simulink model "PEMFuelCellSystem_Before_v01"  (R2025b)
settings: Solver=VariableStepAuto  StartTime=0.0  StopTime=0.1  MaxStep=0.01  RelTol=1e-3  AbsTol=1e-3
model workspace: external: MATLAB File E:\agentwork_pemfc_cEGR_0519\04_Simulink物理网络模型\01_模型\RouteA_GasMixture_Derived\PEMFuelCellSystemWithACustomLibraryParameters.m (data not in the file)
undefined symbols (not defined in the file): anode_tube_D, cathode_tube_D, cegr_valve_max_area, cegr_valve_open_min_area, comp_rpm_TLU, coolant_num_layers, coolant_num_passes, coolant_tube_D, coolant_w_channels, env_p, env_T, env_yH20, env_yO2, radiator_air_area_fins, radiator_air_area_primary, radiator_eta_fin, radiator_N_tubes, radiator_rho, radiator_t_wall, radiator_tube_H, radiator_W, routeA_air_pid_Ki, routeA_air_pid_Kp, routeA_anode_inlet_pressure_MPa_abs, routeA_anode_purge_off_n2_mole_fraction, routeA_anode_purge_on_n2_mole_fraction, routeA_anode_recirculation_base_command, routeA_anode_recirculation_current_gain_A_inv, routeA_anode_rh_setpoint, routeA_cathode_humidifier_gain, routeA_cathode_rh_setpoint, routeA_compressor_cmd_direct, routeA_egr_control_Ki_area, routeA_egr_control_Kp_area, routeA_egr_target_input_mode_id, routeA_egr_valve_actuator_tau, routeA_egr_valve_area_direct, routeA_stack_temperature_set_C, routeA_target_egr_ratio_comp_in, routeA_target_mdot_comp_inlet, routeA_target_oer, routeA_target_p_ca_out_MPa, routeA_voltage_current_max_A, routeA_voltage_current_min_A, routeA_voltage_pi_Ki, routeA_voltage_pi_Kp, stack_area, stack_iL, stack_mea_rho, stack_num_cells, stack_num_channels, stack_t_gdl, stack_t_membrane, stack_w_channels, tank_yH2
libraries: fl_lib x63, FuelCell_lib x53, nesl_utility x42, slpidlib x5
(part 6 of 6)

== system PEMFuelCellSystem_Before_v01/System_Control_Observability/Electrical Load/Inputs/Power Demand ==
  From Workspace : FromWorkspace  VariableName=[drive_cycle_time, drive_cycle_power]
  PS Divide : fl_lib/Physical Signals/Functions/PS Divide
  PS-Simulink Converter : nesl_utility/PS-Simulink Converter  PhysicalDomain=network_engine_domain  SubClassName=ps_output  LeftPortType=input  RightPortType=output  PseudoPeriodic=off  Frequencies=[]  VectorFormat=1-D array  Unit=V  AffineConversion=off
  PS-Simulink Converter1 : nesl_utility/PS-Simulink Converter  PhysicalDomain=network_engine_domain  SubClassName=ps_output  LeftPortType=input  RightPortType=output  PseudoPeriodic=off  Frequencies=[]  VectorFormat=1-D array  Unit=A  AffineConversion=off
  Power Current Limit : fl_lib/Physical Signals/Nonlinear Operators/PS Saturation  upper_limit=routeA_voltage_current_max_A A  lower_limit=routeA_voltage_current_min_A A  ZeroCross=true
  Power kW to W : Gain  Gain=1000
  Simulink-PS Converter : nesl_utility/Simulink-PS Converter  PhysicalDomain=network_engine_domain  SubClassName=ps_input  LeftPortType=input  RightPortType=output  PseudoPeriodic=off  Frequencies=[]  NoiseDistribution=none  NoiseParameters=[]  Unit=W  AffineConversion=off  FilteringAndDerivatives=provide  SimscapeFilterOrder=1  InputFilterTimeConstant=0.001  UdotUserProvided=0
  i : PMIOPort  Side=Left
  v : PMIOPort  Port=2  Side=Left
  tag scope: i_stack=global, v_stack=global
  wires:
  PS-Simulink Converter1/1 -> [i_stack]  "routeA_power_current_cmd_limited_A"
  PS-Simulink Converter/1 -> [v_stack]
  From Workspace/1 -> Power kW to W/1
  Power kW to W/1 -> Simulink-PS Converter/1
  connections:
  PS-Simulink Converter1/LConn1 -- Power Current Limit/RConn1 -- i/RConn1
  v/RConn1 -- PS-Simulink Converter/LConn1 -- PS Divide/LConn2
  PS Divide/LConn1 -- Simulink-PS Converter/RConn1
  PS Divide/RConn1 -- Power Current Limit/LConn1

== system PEMFuelCellSystem_Before_v01/System_Control_Observability/Electrical Load/Inputs/Voltage Demand ==
  Current Command : nesl_utility/Simulink-PS Converter  PhysicalDomain=network_engine_domain  SubClassName=ps_input  LeftPortType=input  RightPortType=output  PseudoPeriodic=off  Frequencies=[]  NoiseDistribution=none  NoiseParameters=[]  Unit=A  AffineConversion=off  FilteringAndDerivatives=provide  SimscapeFilterOrder=1  InputFilterTimeConstant=0.001  UdotUserProvided=0
  Current Command Dynamics : TransferFcn  Denominator=[0.1 1]
  Raw PI Diagnostic : slpidlib/PID Controller  Controller=PI  Form=Parallel  TimeDomain=Continuous-time  UseExternalTs=off  SampleTime=-1  IntegratorMethod=Forward Euler  FilterMethod=Forward Euler  ControllerParametersSource=internal  P=routeA_voltage_pi_Kp  I=routeA_voltage_pi_Ki  UseKiTs=off  D=0  UseExternalDerivativeSource=off  N=100  UseFilter=on  TunerSelectOption=Transfer Function Based (PID Tuner App)  InitialConditionSource=internal  InitialConditionForIntegrator=0  InitialConditionForFilter=0  DifferentiatorICPrevScaledInput=0  ExternalReset=none  TrackingMode=off  Kt=1  LimitOutput=off  SatLimitsSource=internal  UpperSaturationLimit=inf  LowerSaturationLimit=-inf  LinearizeAsGain=on  AntiWindupMode=none  Kb=1  LimitIntegrator=off  UpperIntegratorSaturationLimit=inf  LowerIntegratorSaturationLimit=-inf  POutMin=[]  POutMax=[]  IOutMin=[]  IOutMax=[]  DOutMin=[]  DOutMax=[]  NOutMin=[]  NOutMax=[]  SumOutMin=[]  SumOutMax=[]  SaturationOutMin=[]  SaturationOutMax=[]  PParamMin=[]  PParamMax=[]  IParamMin=[]  IParamMax=[]  DParamMin=[]  DParamMax=[]  NParamMin=[]  NParamMax=[]  KbParamMin=[]  KbParamMax=[]  KtParamMin=[]  KtParamMax=[]  KbOutMin=[]  KbOutMax=[]  KtOutMin=[]  KtOutMax=[]  IntegratorOutMin=[]  IntegratorOutMax=[]  FilterOutMin=[]  FilterOutMax=[]  SumI1OutMin=[]  SumI1OutMax=[]  SumI2OutMin=[]  SumI2OutMax=[]  SumI3OutMin=[]  SumI3OutMax=[]  SumI4OutMin=[]  SumI4OutMax=[]  SumDOutMin=[]  SumDOutMax=[]  DifferentiatorOutMin=[]  DifferentiatorOutMax=[]  FilterDiffOutCoefMin=[]  FilterDiffOutCoefMax=[]  ReciprocalOutMin=[]  ReciprocalOutMax=[]  SumDenOutMin=[]  SumDenOutMax=[]  SumNumOutMin=[]  SumNumOutMax=[]  DivideOutMin=[]  DivideOutMax=[]  UdiffTsProdOutMin=[]  UdiffTsProdOutMax=[]  NTsProdOutMin=[]  NTsProdOutMax=[]  UintegralTsProdOutMin=[]  UintegralTsProdOutMax=[]  UngainTsProdOutMin=[]  UngainTsProdOutMax=[]  ClampingZeroOutDataTypeStr=Inherit: Inherit via back propagation  ClampingZeroOutMin=[]  ClampingZeroOutMax=[]  FilterDenConstantOutDataTypeStr=Inherit: Inherit via back propagation  FilterDenConstantOutMin=[]  FilterDenConstantOutMax=[]  PCopyOutDataTypeStr=Inherit: Inherit via back propagation  PCopyOutMin=[]  PCopyOutMax=[]  NCopyOutDataTypeStr=Inherit: Inherit via back propagation  NCopyOutMin=[]  NCopyOutMax=[]  IntegratorContinuousStateAttributes=''  IntegratorStateMustResolveToSignalObject=off  IntegratorRTWStateStorageClass=Auto  FilterContinuousStateAttributes=''  FilterStateMustResolveToSignalObject=off  FilterRTWStateStorageClass=Auto  ParallelPVariant=InternalParameters  IdealPVariant=Disabled  IVariant=InternalParameters  DVariant=Disabled  IntegratorVariant=Continuous  SatVariant=Disabled  AWVariant=Passthrough  PCopyVariant=Disabled  TRVariant=Disabled  FdbkBlocksVariant=Forward  IdealPFdbkVariant=Disabled  SatFdbkVariant=Disabled  DerivativeFilterVariant=Disabled  NVariant=Disabled  NCopyVariant=Disabled_SignalSpec  FilterICVariant=Disabled  IntegratorICVariant=InternalICs  ExternalResetVariant=Disabled  TRSumVariant=Passthrough  SumFdbkVariant=Disabled  SumVariant=Sum_PI  TsampFilterVariant=InternalTs  TsampNgainVariant=Passthrough  TsampIntegralVariant=Disabled_SignalSpec  ExternalSaturationOutDataTypeStr=Inherit: Same as second input  DerivativeSourceVariant=Disabled  PreIntVariant=InternalPreInt
  Saturation Status : RelationalOperator  Operator=~=
  Saturation Status Terminator : Terminator
  Voltage Error : Sum  Inputs=+-
  Voltage Measurement : nesl_utility/PS-Simulink Converter  PhysicalDomain=network_engine_domain  SubClassName=ps_output  LeftPortType=input  RightPortType=output  PseudoPeriodic=off  Frequencies=[]  VectorFormat=inherit  Unit=V  AffineConversion=off
  Voltage PI : slpidlib/PID Controller  Controller=PI  Form=Parallel  TimeDomain=Continuous-time  UseExternalTs=off  SampleTime=-1  IntegratorMethod=Forward Euler  FilterMethod=Forward Euler  ControllerParametersSource=internal  P=routeA_voltage_pi_Kp  I=routeA_voltage_pi_Ki  UseKiTs=off  D=0  UseExternalDerivativeSource=off  N=100  UseFilter=on  TunerSelectOption=Transfer Function Based (PID Tuner App)  InitialConditionSource=internal  InitialConditionForIntegrator=0  InitialConditionForFilter=0  DifferentiatorICPrevScaledInput=0  ExternalReset=none  TrackingMode=off  Kt=1  LimitOutput=on  SatLimitsSource=internal  UpperSaturationLimit=routeA_voltage_current_max_A  LowerSaturationLimit=routeA_voltage_current_min_A  LinearizeAsGain=on  AntiWindupMode=clamping  Kb=1  LimitIntegrator=off  UpperIntegratorSaturationLimit=inf  LowerIntegratorSaturationLimit=-inf  POutMin=[]  POutMax=[]  IOutMin=[]  IOutMax=[]  DOutMin=[]  DOutMax=[]  NOutMin=[]  NOutMax=[]  SumOutMin=[]  SumOutMax=[]  SaturationOutMin=[]  SaturationOutMax=[]  PParamMin=[]  PParamMax=[]  IParamMin=[]  IParamMax=[]  DParamMin=[]  DParamMax=[]  NParamMin=[]  NParamMax=[]  KbParamMin=[]  KbParamMax=[]  KtParamMin=[]  KtParamMax=[]  KbOutMin=[]  KbOutMax=[]  KtOutMin=[]  KtOutMax=[]  IntegratorOutMin=[]  IntegratorOutMax=[]  FilterOutMin=[]  FilterOutMax=[]  SumI1OutMin=[]  SumI1OutMax=[]  SumI2OutMin=[]  SumI2OutMax=[]  SumI3OutMin=[]  SumI3OutMax=[]  SumI4OutMin=[]  SumI4OutMax=[]  SumDOutMin=[]  SumDOutMax=[]  DifferentiatorOutMin=[]  DifferentiatorOutMax=[]  FilterDiffOutCoefMin=[]  FilterDiffOutCoefMax=[]  ReciprocalOutMin=[]  ReciprocalOutMax=[]  SumDenOutMin=[]  SumDenOutMax=[]  SumNumOutMin=[]  SumNumOutMax=[]  DivideOutMin=[]  DivideOutMax=[]  UdiffTsProdOutMin=[]  UdiffTsProdOutMax=[]  NTsProdOutMin=[]  NTsProdOutMax=[]  UintegralTsProdOutMin=[]  UintegralTsProdOutMax=[]  UngainTsProdOutMin=[]  UngainTsProdOutMax=[]  ClampingZeroOutDataTypeStr=Inherit: Inherit via back propagation  ClampingZeroOutMin=[]  ClampingZeroOutMax=[]  FilterDenConstantOutDataTypeStr=Inherit: Inherit via back propagation  FilterDenConstantOutMin=[]  FilterDenConstantOutMax=[]  PCopyOutDataTypeStr=Inherit: Inherit via back propagation  PCopyOutMin=[]  PCopyOutMax=[]  NCopyOutDataTypeStr=Inherit: Inherit via back propagation  NCopyOutMin=[]  NCopyOutMax=[]  IntegratorContinuousStateAttributes=''  IntegratorStateMustResolveToSignalObject=off  IntegratorRTWStateStorageClass=Auto  FilterContinuousStateAttributes=''  FilterStateMustResolveToSignalObject=off  FilterRTWStateStorageClass=Auto  ParallelPVariant=InternalParameters  IdealPVariant=Disabled  IVariant=InternalParameters  DVariant=Disabled  IntegratorVariant=Continuous  SatVariant=Enabled  AWVariant=ContClampingParallel  PCopyVariant=Disabled  TRVariant=Disabled  FdbkBlocksVariant=Forward  IdealPFdbkVariant=Disabled  SatFdbkVariant=Disabled  DerivativeFilterVariant=Disabled  NVariant=Disabled  NCopyVariant=Disabled_SignalSpec  FilterICVariant=Disabled  IntegratorICVariant=InternalICs  ExternalResetVariant=Disabled  TRSumVariant=Passthrough  SumFdbkVariant=Disabled  SumVariant=Sum_PI  TsampFilterVariant=InternalTs  TsampNgainVariant=Passthrough  TsampIntegralVariant=Disabled_SignalSpec  ExternalSaturationOutDataTypeStr=Inherit: Same as second input  DerivativeSourceVariant=Disabled  PreIntVariant=InternalPreInt
  Voltage Reference : FromWorkspace  VariableName=[drive_cycle_time, drive_cycle_voltage]
  i : PMIOPort  Side=Left
  v : PMIOPort  Port=2  Side=Left
  tag scope: i_stack=global, v_stack=global
  wires:
  Current Command Dynamics/1 -> [i_stack], Current Command/1  "routeA_voltage_current_cmd_A"
  Voltage PI/1 -> Current Command Dynamics/1, Saturation Status/2  "routeA_voltage_current_cmd_limited_A"
  Voltage Error/1 -> Raw PI Diagnostic/1, Voltage PI/1  "routeA_voltage_control_error_V"
  Voltage Reference/1 -> Voltage Error/2  "routeA_voltage_ref_V"
  Voltage Measurement/1 -> Voltage Error/1, [v_stack]
  Raw PI Diagnostic/1 -> Saturation Status/1  "routeA_voltage_current_cmd_raw_A"
  Saturation Status/1 -> Saturation Status Terminator/1  "routeA_voltage_current_saturated"
  connections:
  v/RConn1 -- Voltage Measurement/LConn1
  Current Command/RConn1 -- i/RConn1

== matlab function PEMFuelCellSystem_Before_v01/Cathode_Exhaust_Backpressure_Water/SeparatorOrCondensation ==
  data: p_MPa input; m_water_sep output; T_degC input; y_i input; egr_mdot input; exhaust_mdot input
function m_water_sep = SeparatorOrCondensation(p_MPa,T_degC,y_i,egr_mdot,exhaust_mdot)
%#codegen
% L2 saturation-excess estimator. Source: l2_saturation_excess_estimator.
p = max(double(p_MPa), 1e-6);
T = double(T_degC);
if T > 200
    Tc = T - 273.15;
else
    Tc = T;
end
Tc = min(max(Tc, -40), 120);
if numel(y_i) >= 4
    yH2O = max(double(y_i(4)), 0);
else
    yH2O = 0;
end
pSat_kPa = 0.61121 * exp((18.678 - Tc/234.5) * (Tc/(257.14 + Tc)));
pSat_MPa = max(pSat_kPa * 1e-3, 1e-9);
ySat = min(max(pSat_MPa / p, 0), 1);
excess = max(yH2O - ySat, 0);
mdotTotal = max(double(egr_mdot), 0) + max(double(exhaust_mdot), 0);
m_water_sep = mdotTotal * excess;
end
